simulink model "simulimnk_motor"  (R2021a)
settings: Solver=VariableStepAuto  StartTime=0.0  StopTime=10.0  RelTol=1e-3
undefined symbols (not defined in the file or in its folder): K
libraries: simulink x2
settings Model: Creator=paige  LastModifiedBy=paige

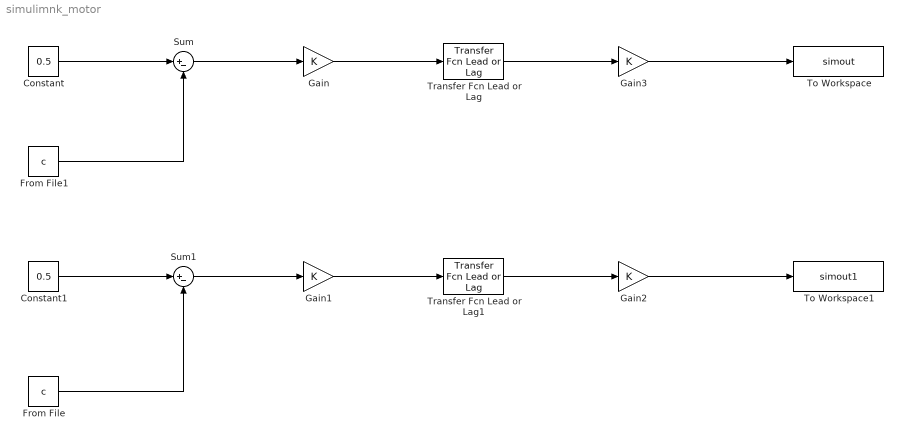
== system simulimnk_motor ==
  Constant : Constant  Value=0.5
  Constant1 : Constant  Value=0.5
  From File : FromFile  FileName=c  SampleTime=0
  From File1 : FromFile  FileName=c  SampleTime=0
  Gain{,1..3} (4 alike) : Gain  Gain=K
      Gain2 settings: AttributesFormatString=pi/180
      Gain3 settings: AttributesFormatString=pi/180
  Sum : Sum  Inputs=|+-
  Sum1 : Sum  Inputs=|+-
  To Workspace : ToWorkspace  VariableName=simout  SaveFormat=Timeseries  SampleTime=-1
      settings: AttributesFormatString=send to workspace
  To Workspace1 : ToWorkspace  VariableName=simout1  SaveFormat=Timeseries  SampleTime=-1
      settings: AttributesFormatString=send to workspace
  Transfer Fcn Lead or Lag : simulink/Discrete/Transfer Fcn Lead or Lag  PoleZ=0.95  ZeroZ=0.75  ICPrevOutput=0.0  ICPrevInput=0.0  DoSatur=off
      settings: AttributesFormatString=lead/lag  SourceProductBaseCode=SL
  Transfer Fcn Lead or Lag1 : simulink/Discrete/Transfer Fcn Lead or Lag  PoleZ=0.95  ZeroZ=0.75  ICPrevOutput=0.0  ICPrevInput=0.0  DoSatur=off
      settings: AttributesFormatString=lead/lag  SourceProductBaseCode=SL
  wires:
  Constant/1 -> Sum/1
  From File1/1 -> Sum/2
  Sum/1 -> Gain/1
  Gain/1 -> Transfer Fcn Lead or Lag/1
  Transfer Fcn Lead or Lag/1 -> Gain3/1
  Gain3/1 -> To Workspace/1
  Constant1/1 -> Sum1/1
  From File/1 -> Sum1/2
  Sum1/1 -> Gain1/1
  Gain1/1 -> Transfer Fcn Lead or Lag1/1
  Transfer Fcn Lead or Lag1/1 -> Gain2/1
  Gain2/1 -> To Workspace1/1
